simulink model "thirdBasicFull"  (R2018b)
settings: Solver=FixedStepDiscrete  StartTime=0.0  StopTime=10.0  RelTol=1e-3
settings Model: Creator=matlab  LastModifiedBy=matlab
settings DataIOCC: SaveOutput=off  SignalLogging=off  SaveTime=off
settings OptimizationCC: DefaultParameterBehavior=Inlined  EnhancedBackFolding=on  PassReuseOutputArgsAs=Individual arguments  OptimizeBlockOrder=speed  DifferentSizesBufferReuse=on  OptimizationCustomize=off
settings DebuggingCC: ParameterTunabilityLossMsg=error
settings SFSimCC: MATLABDynamicMemAlloc=off
settings RTWCC: SystemTargetFile=ert.tlc  TemplateMakefile=ert_default_tmf  PostCodeGenCommand=packNGo(buildInfo);  GenerateReport=on  IncludeHyperlinkInReport=on  LaunchReport=on  GenerateTraceInfo=on  GenerateTraceReport=on  GenerateTraceReportSl=on  GenerateTraceReportSf=on  GenerateTraceReportEml=on
settings CodeAppCC: ForceParamTrailComments=on  IgnoreCustomStorageClasses=off  OperatorAnnotations=on  SimulinkDataObjDesc=on  SFDataObjDesc=on  InsertBlockDesc=on
settings ERTTargetCC: TargetLangStandard=C99 (ISO)  GenerateSampleERTMain=on  InlinedParameterPlacement=NonHierarchical  ERTCustomFileTemplate=example_file_process.tlc

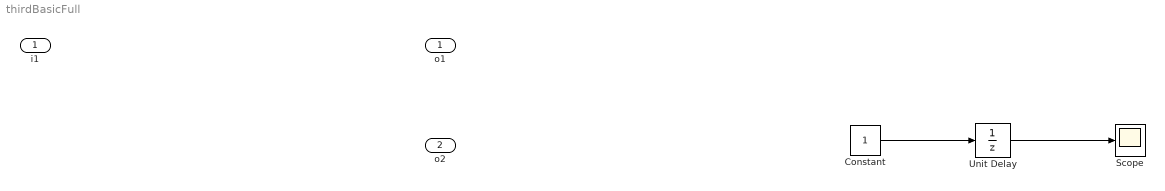
== system thirdBasicFull ==
  i1 : Inport  OutDataTypeStr=MatLab_Boolean  BusOutputAsStruct=on
  Constant : Constant
  Scope : Scope
  Unit Delay : UnitDelay  SampleTime=-1
  o1 : Outport  OutDataTypeStr=MatLab_Boolean
  o2 : Outport  Port=2  OutDataTypeStr=MatLab_Boolean
  wires:
  Constant/1 -> Unit Delay/1
  Unit Delay/1 -> Scope/1
